simulink model "slxfkineDemo"  (R2016a)
settings: Solver=ode5  StartTime=0.0  StopTime=inf  FixedStep=0.001  RelTol=1e-3
libraries: dcpctrl x1
settings Model: SimulationMode=external  Creator=julianleland  LastModifiedBy=julianleland
settings HardwareCC: ProdBitPerLong=64  ProdLargestAtomicFloat=None  ProdHWDeviceType=Intel->x86-64  TargetBitPerLong=64  TargetBitPerPointer=64  TargetIntDivRoundTo=Zero  TargetEndianess=LittleEndian  TargetWordSize=64  TargetHWDeviceType=Intel->x86-64
settings RTWCC: SystemTargetFile=sldrt.tlc  TemplateMakefile=sldrt.tmf  Description=Simulink Desktop Real-Time  RTWCompilerOptimization=on
settings CodeAppCC: MaxIdLength=95
settings SimulinkDesktopRealTimeCC: TargetPreCompLibLocation=/Applications/MATLAB_R2016a.app/toolbox/sldrt/lib/maci64  TargetLangStandard=C89/C90 (ANSI)  SupportVariableSizeSignals=off

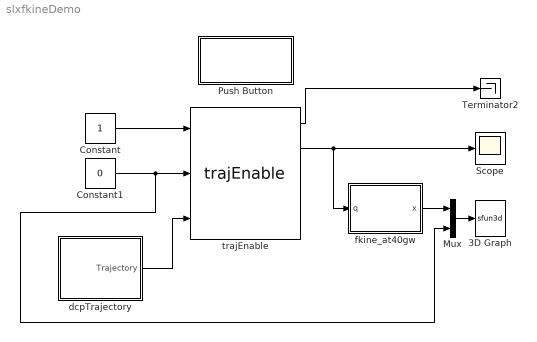
== system slxfkineDemo ==
  3D Graph : S-Function  LoadFcn=if exist('sfun3d','file'), sfun3d([],[],[],'LoadBlock'); end  FunctionName=sfun3d  Parameters=ax,T,np,cp,gd,ls,mk  SFunctionDeploymentMode=off  EnableBusSupport=off  mask(3D Graph){np=1, ax=[2000 6000 -2000 2000 -2000 2000], cp=[6000 -2000 2000], gd=on, ls=-, mk=o, T=-1}
      mask prompts: np "Number of point (lines)"; ax "[xmin xmax  ymin ymax zmin zmax]"; cp "Camera position (use [0 0 1] for 2D XY view)"; gd "Grid (on|off)"; ls "LineStyle"; mk "Marker"; T "Sampling Time"
      mask help:
      | This block plots the position of several points in the XYZ space. The input contains the coordinates of all the points (x1,y1,z1,x2,y2,z2,...).
      | The number of points (lines), the XYZ ranges, camera position, grid, linestyle, marker and sampling time, can be set as mask parameters.
      settings: CopyFcn=if exist('sfun3d','file'), sfun3d([],[],[],'CopyBlock'); end  DeleteFcn=if exist('sfun3d','file'), sfun3d([],[],[],'DeleteBlock'); end  NameChangeFcn=if exist('sfun3d','file'), sfun3d([],[],[],'NameChange'); end
      mask Help:
      | This block plots the position of several points in the XYZ space. The input contains the coordinates of all the points (x1,y1,z1,x2,y2,z2,...).
      | The number of points (lines), the XYZ ranges, camera position, grid, linestyle, marker and sampling time, can be set as mask parameters.
      mask TypeOptions ls: - | -- | : | -. | none
      mask TypeOptions mk: none | . | + | o | * | x | square | diamond | v | ^ | > | < | pentagram | hexagram
      mask Display: plot([.05 .95 .95 .05 .05],[.45 .45 .95 .95 .45], 0.5+cos(0:0.1:2*pi)*0.3,0.7+sin(0:0.1:2*pi)*0.2)
  Constant : Constant
  Constant1 : Constant  Value=0
  Mux : Mux  Inputs=2
  Push Button : Subsystem  DialogController=hmiCreateDDGDialog  IsWebBlock=on  mask(MWDashboardBlock){webBlockId=70571214-1623-4fe4-a991-a5e4601e90b3, webBlockType=pushbutton, ShowInLibBrwoser=on, ShowInitialText=on, HMISrcModelName=slxfkineDemo}
      mask prompts: webBlockId "WebBlock Id"; webBlockType "WebBlock Type"; HMISrcModelName "Source Model"
      mask Help: helpview([docroot '/mapfiles/simulink.map'], 'hmi_push_button')
      mask Display:
      | model = bdroot(gcb);
      | if strcmp(get_param(model,'BlockDiagramType'), 'library')
      |     image([(matlabroot) '/toolbox/simulink/hmi/icons/PushButton.png']);
      | end
  Scope : Scope
  Terminator2 : Terminator
  dcpTrajectory : Subsystem
  fkine_at40gw : MATLAB Function  TreatAsAtomicUnit=on
  trajEnable : dcpctrl/trajEnable
  wires:
  dcpTrajectory/1(Trajectory) -> trajEnable/3
  trajEnable/1 -> Terminator2/1
  Constant1/1 -> Mux/2, trajEnable/2
  trajEnable/2 -> Scope/1, fkine_at40gw/1(q)
  Constant/1 -> trajEnable/1
  fkine_at40gw/1(x) -> Mux/1
  Mux/1 -> 3D Graph/1

== system slxfkineDemo/Push Button ==

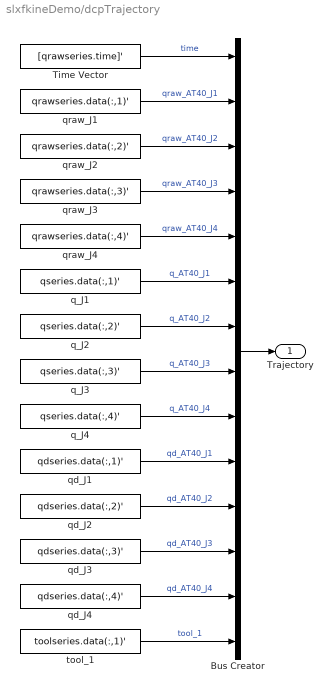
== system slxfkineDemo/dcpTrajectory ==
  Bus Creator : BusCreator  Inputs='time','qraw_AT40_J1','qraw_AT40_J2','qraw_AT40_J3','qraw_AT40_J4','q_AT40_J1','q_AT40_J2','q_AT40_J3','q_AT40_J4','qd_AT40_J1','qd_AT40_J2','qd_AT40_J3','qd_AT40_J4','tool_1'
  Time Vector : FromWorkspace  VariableName=[qrawseries.time]'  SampleTime=0
  q_J1 : FromWorkspace  VariableName=qseries.data(:,1)'  SampleTime=0
  q_J2 : FromWorkspace  VariableName=qseries.data(:,2)'  SampleTime=0
  q_J3 : FromWorkspace  VariableName=qseries.data(:,3)'  SampleTime=0
  q_J4 : FromWorkspace  VariableName=qseries.data(:,4)'  SampleTime=0
  qd_J1 : FromWorkspace  VariableName=qdseries.data(:,1)'  SampleTime=0
  qd_J2 : FromWorkspace  VariableName=qdseries.data(:,2)'  SampleTime=0
  qd_J3 : FromWorkspace  VariableName=qdseries.data(:,3)'  SampleTime=0
  qd_J4 : FromWorkspace  VariableName=qdseries.data(:,4)'  SampleTime=0
  qraw_J1 : FromWorkspace  VariableName=qrawseries.data(:,1)'  SampleTime=0
  qraw_J2 : FromWorkspace  VariableName=qrawseries.data(:,2)'  SampleTime=0
  qraw_J3 : FromWorkspace  VariableName=qrawseries.data(:,3)'  SampleTime=0
  qraw_J4 : FromWorkspace  VariableName=qrawseries.data(:,4)'  SampleTime=0
  tool_1 : FromWorkspace  VariableName=toolseries.data(:,1)'  SampleTime=0
  Trajectory : Outport
  wires:
  tool_1/1 -> Bus Creator/14  "tool_1"
  Bus Creator/1 -> Trajectory/1
  qraw_J4/1 -> Bus Creator/5  "qraw_AT40_J4"
  qraw_J2/1 -> Bus Creator/3  "qraw_AT40_J2"
  Time Vector/1 -> Bus Creator/1  "time"
  qraw_J3/1 -> Bus Creator/4  "qraw_AT40_J3"
  qraw_J1/1 -> Bus Creator/2  "qraw_AT40_J1"
  q_J1/1 -> Bus Creator/6  "q_AT40_J1"
  q_J2/1 -> Bus Creator/7  "q_AT40_J2"
  q_J3/1 -> Bus Creator/8  "q_AT40_J3"
  q_J4/1 -> Bus Creator/9  "q_AT40_J4"
  qd_J1/1 -> Bus Creator/10  "qd_AT40_J1"
  qd_J2/1 -> Bus Creator/11  "qd_AT40_J2"
  qd_J3/1 -> Bus Creator/12  "qd_AT40_J3"
  qd_J4/1 -> Bus Creator/13  "qd_AT40_J4"

== matlab function slxfkineDemo/fkine_at40gw ==
  data: q input; x output
function x = fcn(q)
%#codegen

x_temp = fkine_at40gw(q(1),q(2),q(3),q(4))*[1;0;0;0];
x = x_temp(2:4);
